simulink model "fourier_series_31"  (R2018a)
settings: Solver=VariableStepAuto  StartTime=0.0  StopTime=10  RelTol=1e-3
libraries: simulink x1
settings Model: Creator=barne  LastModifiedBy=weishij2

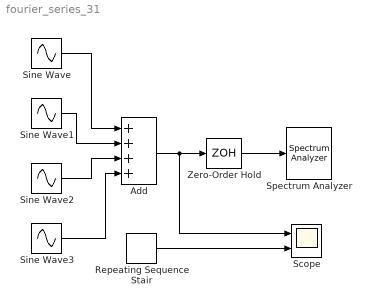
== system fourier_series_31 ==
  Add : Sum  Inputs=++++
  Repeating Sequence Stair : simulink/Sources/Repeating Sequence Stair  OutValues=[-1 1]  tsamp=1/64  OutMin=[]  OutMax=[]  OutDataTypeStr=double  OutputDataTypeScalingMode=double  OutDataType=fixdt(0,8)  ConRadixGroup=Best Precision: Vector-wise  OutScaling=2^-12
  Scope : Scope  NumInputPorts=2
  Sine Wave : Sin  Amplitude=(4/pi)*(1/1)  Frequency=2*pi*1*32  SampleTime=0
  Sine Wave1 : Sin  Amplitude=(4/pi)*(1/3)  Frequency=2*pi*3*32  SampleTime=0
  Sine Wave2 : Sin  Amplitude=(4/pi)*(1/5)  Frequency=2*pi*5*32  SampleTime=0
  Sine Wave3 : Sin  Amplitude=(4/pi)*(1/7)  Frequency=2*pi*7*32  SampleTime=0
  Spectrum Analyzer : SpectrumAnalyzer
  Zero-Order Hold : ZeroOrderHold  SampleTime=2^(-10)
  wires:
  Zero-Order Hold/1 -> Spectrum Analyzer/1
  Sine Wave/1 -> Add/1
  Sine Wave1/1 -> Add/2
  Sine Wave2/1 -> Add/3
  Sine Wave3/1 -> Add/4
  Add/1 -> Scope/1, Zero-Order Hold/1
  Repeating Sequence Stair/1 -> Scope/2
